simulink model "DP7_3_Step"  (R2019b)
settings: Solver=VariableStepAuto  StartTime=0.0  StopTime=10.0  RelTol=1e-3
libraries: simulink_extras x1
settings Model: Creator=Shishir  LastModifiedBy=Shishir

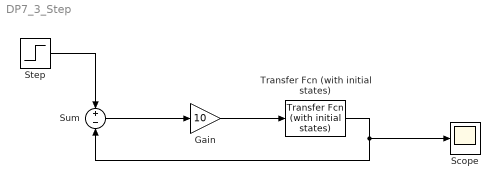
== system DP7_3_Step ==
  Gain : Gain  Gain=10
  Scope : Scope
  Step : Step  Time=0  SampleTime=0
  Sum : Sum  Inputs=+-
  Transfer Fcn (with initial states) : simulink_extras/Additional Linear/Transfer Fcn (with initial states)  N=[1 6.5 12]  D=[1 3 2 0]  X0=0
  wires:
  Gain/1 -> Transfer Fcn (with initial states)/1
  Sum/1 -> Gain/1
  Transfer Fcn (with initial states)/1 -> Scope/1, Sum/2
  Step/1 -> Sum/1
